simulink model "my_sim"  (Simulink 10.3)
settings: Solver=ode45  StartTime=0.0  StopTime=10  RelTol=1e-3  EnableMultiTasking=on
libraries: simulink x2
settings Model: Creator=ljk  LastModifiedBy=YuTaov5  ExtModeTrigMode=oneshot  ExtModeArmWhenConnect=off
settings DataIOCC: SignalLoggingName=sigsOut
settings OptimizationCC: BooleanDataType=off
settings DebuggingCC: SaveWithParameterizedLinksMsg=none  SignalResolutionControl=TryResolveAllWithWarning  MultiTaskDSMMsg=warning  MultiTaskCondExecSysMsg=none
settings HardwareCC: TargetUnknown=on

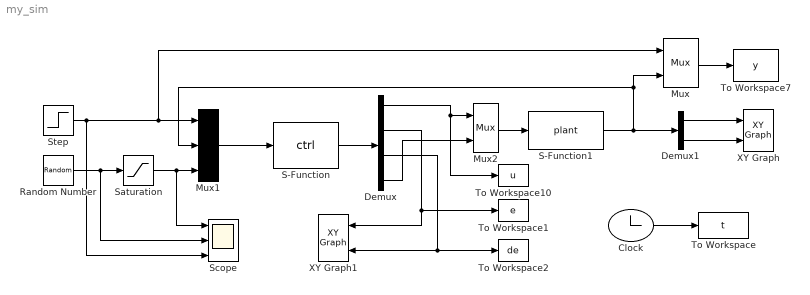
== system my_sim ==
  Clock : Clock
  Demux : Demux
      settings: DisplayOption=none
  Demux1 : Demux  Outputs=2
      settings: DisplayOption=none
  Mux : Mux  Inputs=2
  Mux1 : Mux  Inputs=3
  Mux2 : Mux  Inputs=2
  Random Number : RandomNumber  SampleTime=0.1
  S-Function : S-Function  FunctionName=ctrl  SFunctionDeploymentMode=off  EnableBusSupport=off
  S-Function1 : S-Function  FunctionName=plant  SFunctionDeploymentMode=off  EnableBusSupport=off
  Saturation : Saturate
  Scope : Scope  NumInputPorts=3
  Step : Step  Time=0  SampleTime=0
  To Workspace : ToWorkspace  VariableName=t  SampleTime=-1
  To Workspace1 : ToWorkspace  VariableName=e  SampleTime=-1
  To Workspace10 : ToWorkspace  VariableName=u  SampleTime=-1
  To Workspace2 : ToWorkspace  VariableName=de  SampleTime=-1
  To Workspace7 : ToWorkspace  VariableName=y  SampleTime=-1
  XY Graph : simulink/Sinks/XY Graph  xmin=-1  xmax=1  ymin=-1  ymax=1  st=-1
  XY Graph1 : simulink/Sinks/XY Graph  xmin=-1  xmax=1  ymin=-1  ymax=1  st=-1
  wires:
  Step/1 -> Scope/3, Mux/1, Mux1/1
  Mux1/1 -> S-Function/1
  Clock/1 -> To Workspace/1
  Mux/1 -> To Workspace7/1
  S-Function1/1 -> Mux1/2, Mux/2, Demux1/1
  S-Function/1 -> Demux/1
  Demux/1 -> To Workspace10/1, Mux2/1
  Demux/3 -> XY Graph1/2, To Workspace2/1
  Demux1/1 -> XY Graph/1
  Demux1/2 -> XY Graph/2
  Demux/2 -> To Workspace1/1, XY Graph1/1
  Random Number/1 -> Scope/2, Saturation/1
  Saturation/1 -> Scope/1, Mux1/3
  Demux/4 -> Mux2/2
  Mux2/1 -> S-Function1/1
